simulink model "rajz2"  (R2021a)
settings: Solver=VariableStepAuto  StartTime=0.0  StopTime=10.0  RelTol=1e-3
values from neighbouring files (symbols this model uses):
  A = [-1/2 0 0; 0 0 1; 1 -1 -1]    [maj4.m]
  B = [1;0;0]    [maj4.m]
  C = [0 1 0]    [maj4.m]
  K = acker(A, B, [s1 s2 s3])    [maj4.m]
  Nu = Nxu(end)    [maj4.m]
  Nx = Nxu(1:3)    [maj4.m]
settings Model: Creator=Peti  LastModifiedBy=Peti

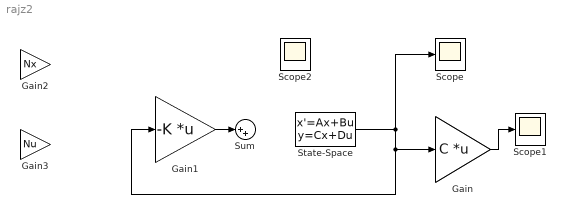
== system rajz2 ==
  Gain : Gain  Gain=C  Multiplication=Matrix(K*u)
  Gain1 : Gain  Gain=-K  Multiplication=Matrix(K*u)
  Gain2 : Gain  Gain=Nx
  Gain3 : Gain  Gain=Nu
  Scope : Scope
  Scope1 : Scope
  Scope2 : Scope
  State-Space : StateSpace  A=A  B=B  C=eye(3)  D=zeros(3,1)  InitialCondition=[1; 0; 0]  ParameterTunability=Unconstrained
  Sum : Sum  Inputs=|++
  wires:
  State-Space/1 -> Gain1/1, Gain/1, Scope/1
  Gain/1 -> Scope1/1
  Gain1/1 -> Sum/1
